simulink model "atan_simulink"  (R2018a)
settings: Solver=FixedStepAuto  StartTime=0.0  StopTime=1000  FixedStep=1  RelTol=1e-3  EnableMultiTasking=on
libraries: hdlsllib x20, simulink x7
settings Model: Creator=john  LastModifiedBy=jjn3896
settings DebuggingCC: SingleTaskRateTransMsg=error
settings CodeAppCC: StateflowObjectComments=on
settings SimscapeCC: SimscapeNormalizeSystem=off

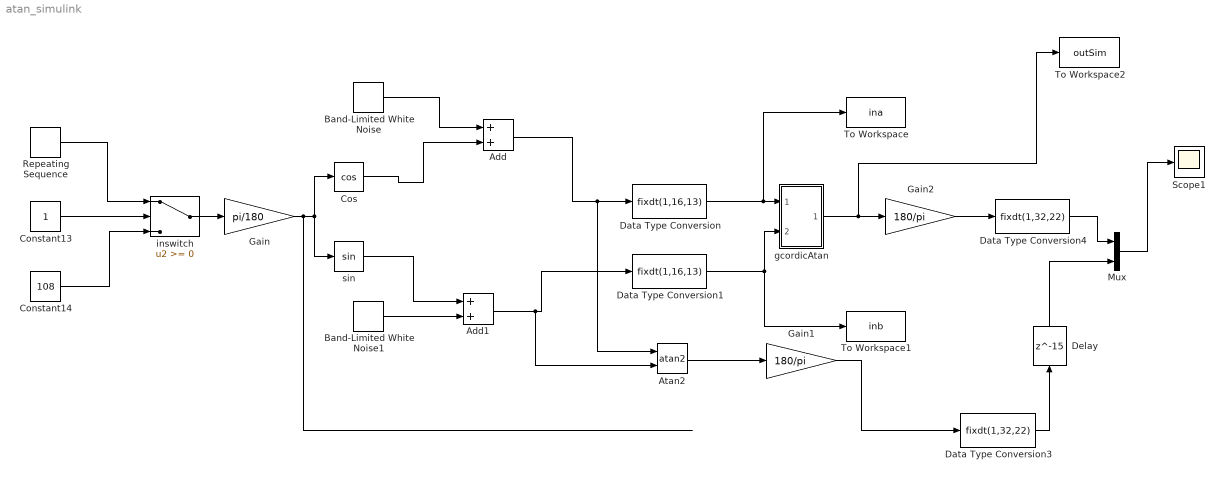
== system atan_simulink ==
  Add : Sum
  Add1 : Sum
  Atan2 : Trigonometry  Operator=atan2
  Band-Limited White Noise : simulink/Sources/Band-Limited White Noise  Cov=[0.1]  Ts=1  seed=[23341]
  Band-Limited White Noise1 : simulink/Sources/Band-Limited White Noise  Cov=[0.1]  Ts=1  seed=[8231]
  Constant13 : Constant
  Constant14 : Constant  Value=108
  Cos : Trigonometry  Operator=cos
  Data Type Conversion : DataTypeConversion  OutDataTypeStr=fixdt(1,16,13)
  Data Type Conversion1 : DataTypeConversion  OutDataTypeStr=fixdt(1,16,13)
  Data Type Conversion3 : DataTypeConversion  OutDataTypeStr=fixdt(1,32,22)
  Data Type Conversion4 : DataTypeConversion  OutDataTypeStr=fixdt(1,32,22)
  Delay : Delay  DelayLength=15
  Gain : Gain  Gain=pi/180
  Gain1 : Gain  Gain=180/pi
  Gain2 : Gain  Gain=180/pi
  Mux : Mux  Inputs=2
  Repeating Sequence : simulink/Sources/Repeating Sequence  rep_seq_t=[0:1:1000]  rep_seq_y=[-180:(360/1000):180]
  Scope1 : Scope
  To Workspace : ToWorkspace  VariableName=ina  SampleTime=-1
      settings: Save2DSignal=2-D array (concatenate along first dimension)
  To Workspace1 : ToWorkspace  VariableName=inb  SampleTime=-1
      settings: Save2DSignal=2-D array (concatenate along first dimension)
  To Workspace2 : ToWorkspace  VariableName=outSim  SampleTime=-1
      settings: Save2DSignal=2-D array (concatenate along first dimension)
  gcordicAtan : Subsystem
  "inswitch " : Switch
  "sin " : Trigonometry
  wires:
  Gain/1 -> Cos/1, "sin "/1
  Mux/1 -> Scope1/1
  "inswitch "/1 -> Gain/1
  gcordicAtan/1(Out1) -> To Workspace2/1, Gain2/1
  Constant13/1 -> "inswitch "/2
  Repeating Sequence/1 -> "inswitch "/1
  Constant14/1 -> "inswitch "/3
  Data Type Conversion/1 -> gcordicAtan/1(In1), To Workspace/1
  Data Type Conversion1/1 -> gcordicAtan/2(In2), To Workspace1/1
  Data Type Conversion3/1 -> Delay/1
  Delay/1 -> Mux/2
  Data Type Conversion4/1 -> Mux/1
  Gain2/1 -> Data Type Conversion4/1
  Band-Limited White Noise/1 -> Add/1
  Band-Limited White Noise1/1 -> Add1/2
  "sin "/1 -> Add1/1
  Cos/1 -> Add/2
  Add/1 -> Atan2/1, Data Type Conversion/1
  Add1/1 -> Atan2/2, Data Type Conversion1/1
  Atan2/1 -> Gain1/1
  Gain1/1 -> Data Type Conversion3/1

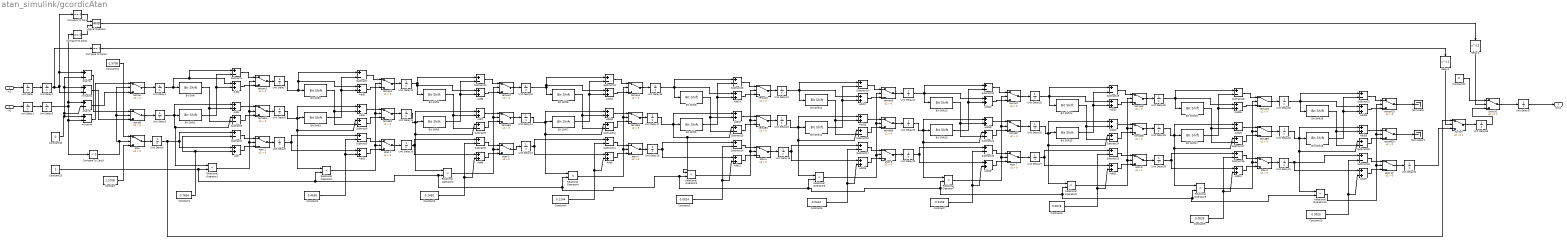
== system atan_simulink/gcordicAtan ==
  In1 : Inport  OutDataTypeStr=fixdt(1,16,13)
  In2 : Inport  Port=2  OutDataTypeStr=fixdt(1,16,13)
  Add{,1..29} (30 alike) : Sum
  Bit Shift : hdlsllib/Logic and Bit Operations/Bit Shift  mode=Shift Right Arithmetic  N=0
      settings: SourceProductName=HDL Coder  SourceProductBaseCode=HD
  Bit Shift1 : hdlsllib/Logic and Bit Operations/Bit Shift  mode=Shift Right Arithmetic  N=0
      settings: SourceProductName=HDL Coder  SourceProductBaseCode=HD
  Bit Shift10 : hdlsllib/Logic and Bit Operations/Bit Shift  mode=Shift Right Arithmetic  N=5
      settings: SourceProductName=HDL Coder  SourceProductBaseCode=HD
  Bit Shift11 : hdlsllib/Logic and Bit Operations/Bit Shift  mode=Shift Right Arithmetic  N=5
      settings: SourceProductName=HDL Coder  SourceProductBaseCode=HD
  Bit Shift12 : hdlsllib/Logic and Bit Operations/Bit Shift  mode=Shift Right Arithmetic  N=6
      settings: SourceProductName=HDL Coder  SourceProductBaseCode=HD
  Bit Shift13 : hdlsllib/Logic and Bit Operations/Bit Shift  mode=Shift Right Arithmetic  N=6
      settings: SourceProductName=HDL Coder  SourceProductBaseCode=HD
  Bit Shift14 : hdlsllib/Logic and Bit Operations/Bit Shift  mode=Shift Right Arithmetic  N=7
      settings: SourceProductName=HDL Coder  SourceProductBaseCode=HD
  Bit Shift15 : hdlsllib/Logic and Bit Operations/Bit Shift  mode=Shift Right Arithmetic  N=7
      settings: SourceProductName=HDL Coder  SourceProductBaseCode=HD
  Bit Shift16 : hdlsllib/Logic and Bit Operations/Bit Shift  mode=Shift Right Arithmetic  N=8
      settings: SourceProductName=HDL Coder  SourceProductBaseCode=HD
  Bit Shift17 : hdlsllib/Logic and Bit Operations/Bit Shift  mode=Shift Right Arithmetic  N=8
      settings: SourceProductName=HDL Coder  SourceProductBaseCode=HD
  Bit Shift18 : hdlsllib/Logic and Bit Operations/Bit Shift  mode=Shift Right Arithmetic  N=9
      settings: SourceProductName=HDL Coder  SourceProductBaseCode=HD
  Bit Shift19 : hdlsllib/Logic and Bit Operations/Bit Shift  mode=Shift Right Arithmetic  N=9
      settings: SourceProductName=HDL Coder  SourceProductBaseCode=HD
  Bit Shift2 : hdlsllib/Logic and Bit Operations/Bit Shift  mode=Shift Right Arithmetic  N=1
      settings: SourceProductName=HDL Coder  SourceProductBaseCode=HD
  Bit Shift3 : hdlsllib/Logic and Bit Operations/Bit Shift  mode=Shift Right Arithmetic  N=1
      settings: SourceProductName=HDL Coder  SourceProductBaseCode=HD
  Bit Shift4 : hdlsllib/Logic and Bit Operations/Bit Shift  mode=Shift Right Arithmetic  N=2
      settings: SourceProductName=HDL Coder  SourceProductBaseCode=HD
  Bit Shift5 : hdlsllib/Logic and Bit Operations/Bit Shift  mode=Shift Right Arithmetic  N=2
      settings: SourceProductName=HDL Coder  SourceProductBaseCode=HD
  Bit Shift6 : hdlsllib/Logic and Bit Operations/Bit Shift  mode=Shift Right Arithmetic  N=3
      settings: SourceProductName=HDL Coder  SourceProductBaseCode=HD
  Bit Shift7 : hdlsllib/Logic and Bit Operations/Bit Shift  mode=Shift Right Arithmetic  N=3
      settings: SourceProductName=HDL Coder  SourceProductBaseCode=HD
  Bit Shift8 : hdlsllib/Logic and Bit Operations/Bit Shift  mode=Shift Right Arithmetic  N=4
      settings: SourceProductName=HDL Coder  SourceProductBaseCode=HD
  Bit Shift9 : hdlsllib/Logic and Bit Operations/Bit Shift  mode=Shift Right Arithmetic  N=4
      settings: SourceProductName=HDL Coder  SourceProductBaseCode=HD
  Compare To Zero : simulink/Logic and Bit Operations/Compare To Zero  relop===  OutDataTypeStr=boolean
  Compare To Zero1 : simulink/Logic and Bit Operations/Compare To Zero  relop===  OutDataTypeStr=boolean
  Compare To Zero2 : simulink/Logic and Bit Operations/Compare To Zero  relop===  OutDataTypeStr=boolean
  Compare To Zero3 : simulink/Logic and Bit Operations/Compare To Zero  relop=<  OutDataTypeStr=boolean
  Constant : Constant  Value=1.5708  OutDataTypeStr=fixdt(1,16,13)
  Constant1 : Constant  Value=0.7854  OutDataTypeStr=fixdt(1,16,13)
  Constant10 : Constant  Value=0.0020  OutDataTypeStr=fixdt(1,16,13)
  Constant11 : Constant  Value=-1.5708  OutDataTypeStr=fixdt(1,16,13)
  Constant12 : Constant  Value=0  OutDataTypeStr=fixdt(1,16,13)
  Constant15 : Constant  Value=0  OutDataTypeStr=fixdt(1,16,13)
  Constant2 : Constant  Value=0.4636  OutDataTypeStr=fixdt(1,16,13)
  Constant23 : Constant  Value=0  OutDataTypeStr=fixdt(1,16,13)
  Constant3 : Constant  Value=0.2450  OutDataTypeStr=fixdt(1,16,13)
  Constant4 : Constant  Value=0.1244  OutDataTypeStr=fixdt(1,16,13)
  Constant5 : Constant  Value=0.0624  OutDataTypeStr=fixdt(1,16,13)
  Constant6 : Constant  Value=0.0312  OutDataTypeStr=fixdt(1,16,13)
  Constant7 : Constant  Value=0.0156  OutDataTypeStr=fixdt(1,16,13)
  Constant8 : Constant  Value=0.0078  OutDataTypeStr=fixdt(1,16,13)
  Constant9 : Constant  Value=0.0039  OutDataTypeStr=fixdt(1,16,13)
  Delay1 : Delay  DelayLength=11
  Delay2 : Delay  DelayLength=12
  Logical Operator : Logic  AllPortsSameDT=off  OutDataTypeStr=boolean
  Relational Operator{1..10} (10 alike) : RelationalOperator  Operator=<  OutDataTypeStr=boolean  RndMeth=Simplest
  Subtract{2..31} (30 alike) : Sum  Inputs=+-
  Switch : Switch  Threshold=1
  Switch1 : Switch  Threshold=1
  Terminator : Terminator
  Terminator1 : Terminator
  Unit Delay{,1..34,56..57} (37 alike) : UnitDelay  SampleTime=-1
  atan {,1..10} (11 alike) : Switch  Criteria=u2 > Threshold
  minusina : Sum  Inputs=+-
  minusinb : Sum  Inputs=+-
  plusina : Sum  Inputs=+-
  "plusinb " : Sum  Inputs=+-
  tempA{,1..10} (11 alike) : Switch  Criteria=u2 > Threshold
  tempB{,1..10} (11 alike) : Switch  Criteria=u2 > Threshold
  Out1 : Outport  OutDataTypeStr=fixdt(1,16,13)
  wires:
  Delay1/1 -> Switch/2
  Switch1/1 -> Unit Delay57/1
  Relational Operator3/1 -> tempA3/2, tempB3/2, atan 3/2
  Relational Operator4/1 -> tempA4/2, tempB4/2, atan 4/2
  Relational Operator6/1 -> tempA6/2, tempB6/2, atan 6/2
  In1/1 -> Unit Delay/1
  Constant23/1 -> Relational Operator10/2, Relational Operator9/2, Relational Operator8/2, Relational Operator7/2, Relational Operator6/2, Relational Operator5/2, Relational Operator4/2, Relational Operator3/2, Relational Operator2/2, Relational Operator1/2
  Constant11/1 -> "atan "/1
  Subtract3/1 -> tempB1/3
  Relational Operator1/1 -> tempA1/2, tempB1/2, atan 1/2
  Relational Operator2/1 -> tempA2/2, tempB2/2, atan 2/2
  In2/1 -> Unit Delay1/1
  Subtract19/1 -> tempA6/1
  Bit Shift12/1 -> Subtract21/2, Add19/2
  Switch/1 -> Unit Delay56/1
  Subtract7/1 -> tempA2/1
  Bit Shift7/1 -> Add11/2, Subtract13/2
  Add12/1 -> atan 5/3
  tempA10/1 -> Terminator/1
  Unit Delay17/1 -> Bit Shift9/1, Relational Operator5/1, Subtract15/1, Add13/1
  Unit Delay29/1 -> Bit Shift17/1, Relational Operator9/1, Subtract27/1, Add25/1
  tempB8/1 -> Unit Delay29/1
  Constant4/1 -> Subtract11/2, Add9/2
  Constant9/1 -> Subtract26/2, Add24/2
  Constant12/1 -> Switch1/1
  Bit Shift13/1 -> Add20/2, Subtract22/2
  atan 4/1 -> Unit Delay16/1
  Compare To Zero/1 -> Logical Operator/1
  Unit Delay27/1 -> Subtract23/1, Add21/1
  Bit Shift16/1 -> Subtract27/2, Add25/2
  Add10/1 -> tempB4/1
  tempA1/1 -> Unit Delay7/1
  Add14/1 -> tempA5/3
  Bit Shift18/1 -> Subtract30/2, Add28/2
  tempA2/1 -> Unit Delay12/1
  Subtract16/1 -> tempA5/1
  atan 8/1 -> Unit Delay28/1
  tempB9/1 -> Unit Delay32/1
  Unit Delay14/1 -> Bit Shift7/1, Relational Operator4/1, Subtract12/1, Add10/1
  tempA5/1 -> Unit Delay21/1
  atan 2/1 -> Unit Delay10/1
  Add8/1 -> tempA3/3
  Unit Delay4/1 -> Add2/1, Subtract4/1, Bit Shift/1
  Relational Operator8/1 -> tempA8/2, tempB8/2, atan 8/2
  Unit Delay15/1 -> Bit Shift6/1, Add11/1, Subtract13/1
  tempA9/1 -> Unit Delay33/1
  Unit Delay31/1 -> Add27/1, Subtract29/1
  Bit Shift14/1 -> Subtract24/2, Add22/2
  Subtract21/1 -> tempB7/3
  Add21/1 -> atan 8/3
  Unit Delay/1 -> Unit Delay2/1
  plusina/1 -> tempB/1
  Unit Delay56/1 -> Switch1/3
  Subtract10/1 -> tempA3/1
  Subtract13/1 -> tempA4/1
  tempA/1 -> Unit Delay4/1
  Add/1 -> atan 1/3
  Unit Delay19/1 -> Subtract17/1, Add15/1
  Unit Delay6/1 -> Switch/1, Add/1, Subtract2/1
  Subtract27/1 -> tempB9/3
  Bit Shift3/1 -> Add5/2, Subtract7/2
  Add20/1 -> tempA7/3
  Constant1/1 -> Subtract2/2, Add/2
  Subtract29/1 -> atan 10/1
  atan 5/1 -> Unit Delay19/1
  Unit Delay34/1 -> Switch/3
  Constant2/1 -> Subtract5/2, Add3/2
  Bit Shift4/1 -> Subtract9/2, Add7/2
  Bit Shift6/1 -> Subtract12/2, Add10/2
  Unit Delay3/1 -> "plusinb "/1, Compare To Zero1/1, minusinb/2, Compare To Zero3/1
  Constant8/1 -> Subtract23/2, Add21/2
  Relational Operator7/1 -> tempA7/2, tempB7/2, atan 7/2
  Unit Delay22/1 -> Subtract20/1, Add18/1
  Bit Shift5/1 -> Add8/2, Subtract10/2
  Constant10/1 -> Subtract29/2, Add27/2
  tempB6/1 -> Unit Delay23/1
  Add28/1 -> tempB10/1
  Bit Shift17/1 -> Add26/2, Subtract28/2
  Logical Operator/1 -> Delay2/1
  Subtract31/1 -> tempA10/1
  Bit Shift/1 -> Subtract3/2, Add1/2
  Unit Delay5/1 -> Relational Operator1/1, Subtract3/1, Add1/1, Bit Shift1/1
  Bit Shift8/1 -> Subtract15/2, Add13/2
  tempB/1 -> Unit Delay5/1
  atan 7/1 -> Unit Delay27/1
  Add7/1 -> tempB3/1
  atan 1/1 -> Unit Delay9/1
  Add11/1 -> tempA4/3
  Unit Delay16/1 -> Subtract14/1, Add12/1
  Compare To Zero3/1 -> tempB/2, tempA/2, "atan "/2
  Subtract15/1 -> tempB5/3
  Unit Delay32/1 -> Bit Shift19/1, Relational Operator10/1, Subtract30/1, Add28/1
  Subtract14/1 -> atan 5/1
  Add15/1 -> atan 6/3
  Unit Delay7/1 -> Add5/1, Subtract7/1, Bit Shift2/1
  Constant3/1 -> Subtract8/2, Add6/2
  Add23/1 -> tempA8/3
  Subtract12/1 -> tempB4/3
  tempB5/1 -> Unit Delay20/1
  Unit Delay20/1 -> Bit Shift11/1, Relational Operator6/1, Subtract18/1, Add16/1
  Add29/1 -> tempA10/3
  Add4/1 -> tempB2/1
  Compare To Zero2/1 -> Delay1/1
  Subtract22/1 -> tempA7/1
  Subtract28/1 -> tempA9/1
  tempA4/1 -> Unit Delay18/1
  Subtract11/1 -> atan 4/1
  Unit Delay33/1 -> Bit Shift18/1, Add29/1, Subtract31/1
  Relational Operator10/1 -> tempA10/2, tempB10/2, atan 10/2
  Subtract23/1 -> atan 8/1
  Bit Shift11/1 -> Add17/2, Subtract19/2
  Delay2/1 -> Switch1/2
  Relational Operator5/1 -> tempA5/2, tempB5/2, atan 5/2
  Constant5/1 -> Subtract14/2, Add12/2
  Add25/1 -> tempB9/1
  "atan "/1 -> Unit Delay6/1
  Add5/1 -> tempA2/3
  Add22/1 -> tempB8/1
  Add18/1 -> atan 7/3
  Constant/1 -> "atan "/3
  Add16/1 -> tempB6/1
  tempB2/1 -> Unit Delay11/1
  Unit Delay21/1 -> Bit Shift10/1, Add17/1, Subtract19/1
  atan 10/1 -> Unit Delay34/1
  Subtract30/1 -> tempB10/3
  Add9/1 -> atan 4/3
  Add1/1 -> tempB1/1
  tempA3/1 -> Unit Delay15/1
  Add27/1 -> atan 10/3
  Unit Delay12/1 -> Bit Shift4/1, Add8/1, Subtract10/1
  atan 3/1 -> Unit Delay13/1
  Subtract2/1 -> atan 1/1
  Unit Delay8/1 -> Bit Shift3/1, Relational Operator2/1, Subtract6/1, Add4/1
  Subtract18/1 -> tempB6/3
  tempB3/1 -> Unit Delay14/1
  Compare To Zero1/1 -> Logical Operator/2
  Unit Delay24/1 -> Bit Shift12/1, Add20/1, Subtract22/1
  Unit Delay23/1 -> Bit Shift13/1, Relational Operator7/1, Subtract21/1, Add19/1
  Unit Delay9/1 -> Subtract5/1, Add3/1
  Subtract17/1 -> atan 6/1
  Add6/1 -> atan 3/3
  tempB7/1 -> Unit Delay26/1
  Subtract20/1 -> atan 7/1
  atan 9/1 -> Unit Delay31/1
  Add13/1 -> tempB5/1
  tempB10/1 -> Terminator1/1
  atan 6/1 -> Unit Delay22/1
  Subtract5/1 -> atan 2/1
  Subtract8/1 -> atan 3/1
  Add24/1 -> atan 9/3
  Add19/1 -> tempB7/1
  Unit Delay28/1 -> Subtract26/1, Add24/1
  Add26/1 -> tempA9/3
  Bit Shift10/1 -> Subtract18/2, Add16/2
  Subtract9/1 -> tempB3/3
  Constant7/1 -> Subtract20/2, Add18/2
  Unit Delay18/1 -> Bit Shift8/1, Add14/1, Subtract16/1
  tempB1/1 -> Unit Delay8/1
  Unit Delay2/1 -> Compare To Zero2/1, minusina/2, plusina/1, Compare To Zero/1
  Unit Delay25/1 -> Bit Shift14/1, Add23/1, Subtract25/1
  Unit Delay26/1 -> Bit Shift15/1, Relational Operator8/1, Subtract24/1, Add22/1
  Relational Operator9/1 -> tempA9/2, tempB9/2, atan 9/2
  Bit Shift2/1 -> Subtract6/2, Add4/2
  Bit Shift9/1 -> Add14/2, Subtract16/2
  Add3/1 -> atan 2/3
  Unit Delay11/1 -> Bit Shift5/1, Relational Operator3/1, Subtract9/1, Add7/1
  Subtract4/1 -> tempA1/1
  tempA8/1 -> Unit Delay30/1
  Add2/1 -> tempA1/3
  Bit Shift1/1 -> Add2/2, Subtract4/2
  Unit Delay1/1 -> Unit Delay3/1
  Bit Shift19/1 -> Add29/2, Subtract31/2
  tempA6/1 -> Unit Delay24/1
  Subtract24/1 -> tempB8/3
  Subtract26/1 -> atan 9/1
  minusina/1 -> tempB/3
  Subtract6/1 -> tempB2/3
  tempA7/1 -> Unit Delay25/1
  "plusinb "/1 -> tempA/3
  Unit Delay13/1 -> Subtract11/1, Add9/1
  Bit Shift15/1 -> Add23/2, Subtract25/2
  minusinb/1 -> tempA/1
  Constant15/1 -> plusina/2, minusina/1, "plusinb "/2, minusinb/1
  Unit Delay30/1 -> Bit Shift16/1, Add26/1, Subtract28/1
  Subtract25/1 -> tempA8/1
  Constant6/1 -> Subtract17/2, Add15/2
  Unit Delay10/1 -> Add6/1, Subtract8/1
  tempB4/1 -> Unit Delay17/1
  Add17/1 -> tempA6/3
  Unit Delay57/1 -> Out1/1
